simulink model "case7"  (R2024b)
settings: Solver=FixedStepAuto  StartTime=0  StopTime=1  FixedStep=1e-7  RelTol=1e-3
values from neighbouring files (symbols this model uses):
  SG_D_1_D = 0.01056    [IEEE9_case_parameters.m]    (also in case1_parameters.m; case2_parameters.m; case3_parameters.m; case4_parameters.m)
  SG_D_1_EnableSaturation = 0    [IEEE9_case_parameters.m]    (also in case1_parameters.m; case2_parameters.m; case3_parameters.m; case4_parameters.m)
  SG_D_1_f0 = 60    [IEEE9_case_parameters.m]    (also in case1_parameters.m; case2_parameters.m; case3_parameters.m; case4_parameters.m)
  SG_D_1_H = 7.5    [IEEE9_case_parameters.m]    (also in case1_parameters.m; case2_parameters.m; case3_parameters.m; case4_parameters.m)
  SG_D_1_K_A = 20    [IEEE9_case_parameters.m]    (also in case1_parameters.m; case2_parameters.m; case3_parameters.m; case4_parameters.m)
  SG_D_1_K_E = 1.000000e+1    (= 10)    [IEEE9_case_parameters.m]    (also in case1_parameters.m; case2_parameters.m; case3_parameters.m; case4_parameters.m)
  SG_D_1_K_F = 2.363    [IEEE9_case_parameters.m]    (also in case1_parameters.m; case2_parameters.m; case3_parameters.m; case4_parameters.m)
  SG_D_1_K_s = 0.5    [IEEE9_case_parameters.m]    (also in case1_parameters.m = 5; case2_parameters.m = 5; case3_parameters.m = 5; case4_parameters.m = 5)
  SG_D_1_R_a = 0.001088    [IEEE9_case_parameters.m]    (also in case1_parameters.m; case2_parameters.m; case3_parameters.m; case4_parameters.m)
  SG_D_1_S_A = 1    [IEEE9_case_parameters.m]    (also in case1_parameters.m; case2_parameters.m; case3_parameters.m; case4_parameters.m)
  SG_D_1_S_B = 0.103    [IEEE9_case_parameters.m]    (also in case1_parameters.m; case2_parameters.m; case3_parameters.m; case4_parameters.m)
  SG_D_1_S_N = 10.659857    [IEEE9_case_parameters.m]    (also in case1_parameters.m; case2_parameters.m; case3_parameters.m; case4_parameters.m)
  SG_D_1_SpeedPara = 200    [IEEE9_case_parameters.m]    (also in case1_parameters.m; case2_parameters.m; case3_parameters.m; case4_parameters.m)
  SG_D_1_T_0 = 0.720173    [IEEE9_case_parameters.m]    (also in case1_parameters.m = 0.755522; case2_parameters.m = 0.808931; case3_parameters.m = 0.869402; case4_parameters.m = 0.729316)
  SG_D_1_T_1 = 0.3    [IEEE9_case_parameters.m]    (also in case1_parameters.m; case2_parameters.m; case3_parameters.m; case4_parameters.m)
  SG_D_1_T_2 = 0.05    [IEEE9_case_parameters.m]    (also in case1_parameters.m; case2_parameters.m; case3_parameters.m; case4_parameters.m)
  SG_D_1_T_3 = 0.02    [IEEE9_case_parameters.m]    (also in case1_parameters.m; case2_parameters.m; case3_parameters.m; case4_parameters.m)
  SG_D_1_T_4 = 0.005    [IEEE9_case_parameters.m]    (also in case1_parameters.m; case2_parameters.m; case3_parameters.m; case4_parameters.m)
  SG_D_1_T_A = 0.02    [IEEE9_case_parameters.m]    (also in case1_parameters.m; case2_parameters.m; case3_parameters.m; case4_parameters.m)
  SG_D_1_T_dd = 8.000000e+0    (= 8)    [IEEE9_case_parameters.m]    (also in case1_parameters.m; case2_parameters.m; case3_parameters.m; case4_parameters.m)
  SG_D_1_T_ddd = 0.04    [IEEE9_case_parameters.m]    (also in case1_parameters.m; case2_parameters.m; case3_parameters.m; case4_parameters.m)
  SG_D_1_T_E = 0.314    [IEEE9_case_parameters.m]    (also in case1_parameters.m; case2_parameters.m; case3_parameters.m; case4_parameters.m)
  SG_D_1_T_F = 0.35    [IEEE9_case_parameters.m]    (also in case1_parameters.m; case2_parameters.m; case3_parameters.m; case4_parameters.m)
  SG_D_1_T_qd = 0.8    [IEEE9_case_parameters.m]    (also in case1_parameters.m; case2_parameters.m; case3_parameters.m; case4_parameters.m)
  SG_D_1_T_qdd = 0.02    [IEEE9_case_parameters.m]    (also in case1_parameters.m; case2_parameters.m; case3_parameters.m; case4_parameters.m)
  SG_D_1_T_speed = 0.1    [IEEE9_case_parameters.m]    (also in case1_parameters.m = 200; case2_parameters.m = 200; case3_parameters.m = 200; case4_parameters.m = 200)
  SG_D_1_T_w = 0.5    [IEEE9_case_parameters.m]    (also in case1_parameters.m; case2_parameters.m; case3_parameters.m; case4_parameters.m)
  SG_D_1_V_ref = 1.990276    [IEEE9_case_parameters.m]    (also in case1_parameters.m = 2.042296; case2_parameters.m = 2.051388; case3_parameters.m = 2.089584; case4_parameters.m = 2.01845)
  SG_D_1_w_ref = 376.991118    [IEEE9_case_parameters.m]    (also in case1_parameters.m; case2_parameters.m; case3_parameters.m; case4_parameters.m)
  SG_D_1_wb = 6.000000e+1    (= 60)    [IEEE9_case_parameters.m]    (also in case1_parameters.m; case2_parameters.m; case3_parameters.m; case4_parameters.m)
  SG_D_1_x_d = 1.9    [IEEE9_case_parameters.m]    (also in case1_parameters.m; case2_parameters.m; case3_parameters.m; case4_parameters.m)
  SG_D_1_x_dd = 0.302    [IEEE9_case_parameters.m]    (also in case1_parameters.m; case2_parameters.m; case3_parameters.m; case4_parameters.m)
  SG_D_1_x_ddd = 0.204    [IEEE9_case_parameters.m]    (also in case1_parameters.m; case2_parameters.m; case3_parameters.m; case4_parameters.m)
  SG_D_1_x_l = 0.05    [IEEE9_case_parameters.m]    (also in case1_parameters.m; case2_parameters.m; case3_parameters.m; case4_parameters.m)
  SG_D_1_x_q = 1.3    [IEEE9_case_parameters.m]    (also in case1_parameters.m; case2_parameters.m; case3_parameters.m; case4_parameters.m)
  SG_D_1_x_qd = 0.5    [IEEE9_case_parameters.m]    (also in case1_parameters.m; case2_parameters.m; case3_parameters.m; case4_parameters.m)
  SG_D_1_x_qdd = 0.3    [IEEE9_case_parameters.m]    (also in case1_parameters.m; case2_parameters.m; case3_parameters.m; case4_parameters.m)
  SG_D_2_D = 0.02    [IEEE9_case_parameters.m]    (also in case1_parameters.m; case2_parameters.m; case3_parameters.m; case4_parameters.m)
  SG_D_2_EnableSaturation = 0    [IEEE9_case_parameters.m]    (also in case1_parameters.m; case2_parameters.m; case3_parameters.m; case4_parameters.m)
  SG_D_2_f0 = 60    [IEEE9_case_parameters.m]    (also in case1_parameters.m; case2_parameters.m; case3_parameters.m; case4_parameters.m)
  SG_D_2_H = 8.000000e+0    (= 8)    [IEEE9_case_parameters.m]    (also in case1_parameters.m; case2_parameters.m; case3_parameters.m; case4_parameters.m)
  SG_D_2_K_A = 20    [IEEE9_case_parameters.m]    (also in case1_parameters.m; case2_parameters.m; case3_parameters.m; case4_parameters.m)
  SG_D_2_K_E = 1.000000e+1    (= 10)    [IEEE9_case_parameters.m]    (also in case1_parameters.m; case2_parameters.m; case3_parameters.m; case4_parameters.m)
  SG_D_2_K_F = 2.363    [IEEE9_case_parameters.m]    (also in case1_parameters.m; case2_parameters.m; case3_parameters.m; case4_parameters.m)
  SG_D_2_K_s = 0.5    [IEEE9_case_parameters.m]    (also in case1_parameters.m = 4; case2_parameters.m = 4; case3_parameters.m = 4; case4_parameters.m = 4)
  SG_D_2_R_a = 0.001088    [IEEE9_case_parameters.m]    (also in case1_parameters.m; case2_parameters.m; case3_parameters.m; case4_parameters.m)
  SG_D_2_S_A = 1    [IEEE9_case_parameters.m]    (also in case1_parameters.m; case2_parameters.m; case3_parameters.m; case4_parameters.m)
  SG_D_2_S_B = 0.103    [IEEE9_case_parameters.m]    (also in case1_parameters.m; case2_parameters.m; case3_parameters.m; case4_parameters.m)
  SG_D_2_S_N = 10.659857    [IEEE9_case_parameters.m]    (also in case1_parameters.m; case2_parameters.m; case3_parameters.m; case4_parameters.m)
  SG_D_2_SpeedPara = 200    [IEEE9_case_parameters.m]    (also in case1_parameters.m; case2_parameters.m; case3_parameters.m; case4_parameters.m)
  SG_D_2_T_0 = 1.632913    [IEEE9_case_parameters.m]    (also in case1_parameters.m = 1.632925; case2_parameters.m = 1.632915; case3_parameters.m = 1.632914; case4_parameters.m = 1.632927)
  SG_D_2_T_1 = 0.2    [IEEE9_case_parameters.m]    (also in case1_parameters.m; case2_parameters.m; case3_parameters.m; case4_parameters.m)
  SG_D_2_T_2 = 0.05    [IEEE9_case_parameters.m]    (also in case1_parameters.m; case2_parameters.m; case3_parameters.m; case4_parameters.m)
  SG_D_2_T_3 = 0.02    [IEEE9_case_parameters.m]    (also in case1_parameters.m; case2_parameters.m; case3_parameters.m; case4_parameters.m)
  SG_D_2_T_4 = 0.005    [IEEE9_case_parameters.m]    (also in case1_parameters.m; case2_parameters.m; case3_parameters.m; case4_parameters.m)
  SG_D_2_T_A = 0.02    [IEEE9_case_parameters.m]    (also in case1_parameters.m; case2_parameters.m; case3_parameters.m; case4_parameters.m)
  SG_D_2_T_dd = 7.9    [IEEE9_case_parameters.m]    (also in case1_parameters.m; case2_parameters.m; case3_parameters.m; case4_parameters.m)
  SG_D_2_T_ddd = 0.04    [IEEE9_case_parameters.m]    (also in case1_parameters.m; case2_parameters.m; case3_parameters.m; case4_parameters.m)
  SG_D_2_T_E = 0.314    [IEEE9_case_parameters.m]    (also in case1_parameters.m; case2_parameters.m; case3_parameters.m; case4_parameters.m)
  SG_D_2_T_F = 0.35    [IEEE9_case_parameters.m]    (also in case1_parameters.m; case2_parameters.m; case3_parameters.m; case4_parameters.m)
  SG_D_2_T_qd = 0.8    [IEEE9_case_parameters.m]    (also in case1_parameters.m; case2_parameters.m; case3_parameters.m; case4_parameters.m)
  SG_D_2_T_qdd = 0.015    [IEEE9_case_parameters.m]    (also in case1_parameters.m; case2_parameters.m; case3_parameters.m; case4_parameters.m)
  SG_D_2_T_speed = 0.1    [IEEE9_case_parameters.m]    (also in case1_parameters.m = 150; case2_parameters.m = 150; case3_parameters.m = 150; case4_parameters.m = 150)
  SG_D_2_T_w = 0.35    [IEEE9_case_parameters.m]    (also in case1_parameters.m; case2_parameters.m; case3_parameters.m; case4_parameters.m)
  SG_D_2_V_ref = 2.58547    [IEEE9_case_parameters.m]    (also in case1_parameters.m = 2.597896; case2_parameters.m = 2.587136; case3_parameters.m = 2.586042; case4_parameters.m = 2.599679)
  SG_D_2_w_ref = 376.991118    [IEEE9_case_parameters.m]    (also in case1_parameters.m; case2_parameters.m; case3_parameters.m; case4_parameters.m)
  SG_D_2_wb = 6.000000e+1    (= 60)    [IEEE9_case_parameters.m]    (also in case1_parameters.m; case2_parameters.m; case3_parameters.m; case4_parameters.m)
  SG_D_2_x_d = 1.8    [IEEE9_case_parameters.m]    (also in case1_parameters.m; case2_parameters.m; case3_parameters.m; case4_parameters.m)
  SG_D_2_x_dd = 0.302    [IEEE9_case_parameters.m]    (also in case1_parameters.m; case2_parameters.m; case3_parameters.m; case4_parameters.m)
  SG_D_2_x_ddd = 0.204    [IEEE9_case_parameters.m]    (also in case1_parameters.m; case2_parameters.m; case3_parameters.m; case4_parameters.m)
  SG_D_2_x_l = 0.05    [IEEE9_case_parameters.m]    (also in case1_parameters.m; case2_parameters.m; case3_parameters.m; case4_parameters.m)
  SG_D_2_x_q = 1.25    [IEEE9_case_parameters.m]    (also in case1_parameters.m; case2_parameters.m; case3_parameters.m; case4_parameters.m)
  SG_D_2_x_qd = 0.5    [IEEE9_case_parameters.m]    (also in case1_parameters.m; case2_parameters.m; case3_parameters.m; case4_parameters.m)
  SG_D_2_x_qdd = 0.3    [IEEE9_case_parameters.m]    (also in case1_parameters.m; case2_parameters.m; case3_parameters.m; case4_parameters.m)
  SG_D_3_D = 0.02    [IEEE9_case_parameters.m]    (also in case1_parameters.m; case2_parameters.m; case3_parameters.m; case4_parameters.m)
  SG_D_3_EnableSaturation = 0    [IEEE9_case_parameters.m]    (also in case1_parameters.m; case2_parameters.m; case3_parameters.m; case4_parameters.m)
  SG_D_3_f0 = 60    [IEEE9_case_parameters.m]    (also in case1_parameters.m; case2_parameters.m; case3_parameters.m; case4_parameters.m)
  SG_D_3_H = 7.7    [IEEE9_case_parameters.m]    (also in case1_parameters.m; case2_parameters.m; case3_parameters.m; case4_parameters.m)
  SG_D_3_K_A = 20    [IEEE9_case_parameters.m]    (also in case1_parameters.m; case2_parameters.m; case3_parameters.m; case4_parameters.m)
  SG_D_3_K_E = 1.000000e+1    (= 10)    [IEEE9_case_parameters.m]    (also in case1_parameters.m; case2_parameters.m; case3_parameters.m; case4_parameters.m)
  SG_D_3_K_F = 2.363    [IEEE9_case_parameters.m]    (also in case1_parameters.m; case2_parameters.m; case3_parameters.m; case4_parameters.m)
  SG_D_3_K_s = 0.2    [IEEE9_case_parameters.m]    (also in case1_parameters.m = 2; case2_parameters.m = 2; case3_parameters.m = 2; case4_parameters.m = 2)
  SG_D_3_R_a = 0.001088    [IEEE9_case_parameters.m]    (also in case1_parameters.m; case2_parameters.m; case3_parameters.m; case4_parameters.m)
  SG_D_3_S_A = 1    [IEEE9_case_parameters.m]    (also in case1_parameters.m; case2_parameters.m; case3_parameters.m; case4_parameters.m)
  SG_D_3_S_B = 0.103    [IEEE9_case_parameters.m]    (also in case1_parameters.m; case2_parameters.m; case3_parameters.m; case4_parameters.m)
  SG_D_3_S_N = 10.659857    [IEEE9_case_parameters.m]    (also in case1_parameters.m; case2_parameters.m; case3_parameters.m; case4_parameters.m)
  SG_D_3_SpeedPara = 200    [IEEE9_case_parameters.m]    (also in case1_parameters.m; case2_parameters.m; case3_parameters.m; case4_parameters.m)
  SG_D_3_T_0 = 0.850788    [IEEE9_case_parameters.m]    (also in case1_parameters.m = 0.850786; case2_parameters.m = 0.850787; case3_parameters.m; case4_parameters.m = 0.850786)
  SG_D_3_T_1 = 0.2    [IEEE9_case_parameters.m]    (also in case1_parameters.m; case2_parameters.m; case3_parameters.m; case4_parameters.m)
  SG_D_3_T_2 = 0.05    [IEEE9_case_parameters.m]    (also in case1_parameters.m; case2_parameters.m; case3_parameters.m; case4_parameters.m)
  SG_D_3_T_3 = 0.02    [IEEE9_case_parameters.m]    (also in case1_parameters.m; case2_parameters.m; case3_parameters.m; case4_parameters.m)
  SG_D_3_T_4 = 0.005    [IEEE9_case_parameters.m]    (also in case1_parameters.m; case2_parameters.m; case3_parameters.m; case4_parameters.m)
  SG_D_3_T_A = 0.02    [IEEE9_case_parameters.m]    (also in case1_parameters.m; case2_parameters.m; case3_parameters.m; case4_parameters.m)
  SG_D_3_T_dd = 8.1    [IEEE9_case_parameters.m]    (also in case1_parameters.m; case2_parameters.m; case3_parameters.m; case4_parameters.m)
  SG_D_3_T_ddd = 0.04    [IEEE9_case_parameters.m]    (also in case1_parameters.m; case2_parameters.m; case3_parameters.m; case4_parameters.m)
  SG_D_3_T_E = 0.314    [IEEE9_case_parameters.m]    (also in case1_parameters.m; case2_parameters.m; case3_parameters.m; case4_parameters.m)
  SG_D_3_T_F = 0.35    [IEEE9_case_parameters.m]    (also in case1_parameters.m; case2_parameters.m; case3_parameters.m; case4_parameters.m)
  SG_D_3_T_qd = 0.8    [IEEE9_case_parameters.m]    (also in case1_parameters.m; case2_parameters.m; case3_parameters.m; case4_parameters.m)
  SG_D_3_T_qdd = 0.015    [IEEE9_case_parameters.m]    (also in case1_parameters.m; case2_parameters.m; case3_parameters.m; case4_parameters.m)
  SG_D_3_T_speed = 0.1    [IEEE9_case_parameters.m]    (also in case1_parameters.m = 180; case2_parameters.m = 180; case3_parameters.m = 180; case4_parameters.m = 180)
  SG_D_3_T_w = 0.4    [IEEE9_case_parameters.m]    (also in case1_parameters.m; case2_parameters.m; case3_parameters.m; case4_parameters.m)
  SG_D_3_V_ref = 1.892727    [IEEE9_case_parameters.m]    (also in case1_parameters.m = 1.906439; case2_parameters.m = 1.895535; case3_parameters.m = 1.892105; case4_parameters.m = 1.906598)
  SG_D_3_w_ref = 376.991118    [IEEE9_case_parameters.m]    (also in case1_parameters.m; case2_parameters.m; case3_parameters.m; case4_parameters.m)
  SG_D_3_wb = 6.000000e+1    (= 60)    [IEEE9_case_parameters.m]    (also in case1_parameters.m; case2_parameters.m; case3_parameters.m; case4_parameters.m)
  SG_D_3_x_d = 1.85    [IEEE9_case_parameters.m]    (also in case1_parameters.m; case2_parameters.m; case3_parameters.m; case4_parameters.m)
  SG_D_3_x_dd = 0.302    [IEEE9_case_parameters.m]    (also in case1_parameters.m; case2_parameters.m; case3_parameters.m; case4_parameters.m)
  SG_D_3_x_ddd = 0.204    [IEEE9_case_parameters.m]    (also in case1_parameters.m; case2_parameters.m; case3_parameters.m; case4_parameters.m)
  SG_D_3_x_l = 0.05    [IEEE9_case_parameters.m]    (also in case1_parameters.m; case2_parameters.m; case3_parameters.m; case4_parameters.m)
  SG_D_3_x_q = 1.2    [IEEE9_case_parameters.m]    (also in case1_parameters.m; case2_parameters.m; case3_parameters.m; case4_parameters.m)
  SG_D_3_x_qd = 0.5    [IEEE9_case_parameters.m]    (also in case1_parameters.m; case2_parameters.m; case3_parameters.m; case4_parameters.m)
  SG_D_3_x_qdd = 0.3    [IEEE9_case_parameters.m]    (also in case1_parameters.m; case2_parameters.m; case3_parameters.m; case4_parameters.m)
(part 8 of 12)

== system case7/SG_D_2/d_psi_d_SG_D_2_block ==
  note: d_psi_d_SG_D_2 in case7
      | $2\,\pi \,f_{0}\,\left(v_{d,\mathrm{SG},D,2}\,\sin\left(\theta _{\mathrm{SG},D,2}\right)-v_{q,\mathrm{SG},D,2}\,\cos\left(\theta _{\mathrm{SG},D,2}\right)+\frac{R_{a}\,\left(\frac{\psi _{\mathrm{1d},\mathrm{SG},D,2}\,\left(x_{\mathrm{dd}}-x_{\mathrm{ddd}}\right)}{x_{\mathrm{dd}}-x_{l}}-\psi _{d,\mathrm{SG},D,2}+\frac{\psi _{\mathrm{fd},\mathrm{SG},D,2}\,\left(x_{\mathrm{ddd}}-x_{l}\right)}{x_{\mathrm{dd}}-x_{l}}\right)}{x_{\mathrm{ddd}}}+\frac{\psi _{q,\mathrm{SG},D,2}\,w_{\mathrm{SG},D,2}}{2\,f_{0}\,\pi }\right)$
      | Automatically generated on 2025-10-31 19:24:13 .
  State_psi_1d_SG_D_2_39a46 : Inport
  State_psi_d_SG_D_2_1ecaf : Inport  Port=2
  State_psi_fd_SG_D_2_079ef : Inport  Port=3
  Input_v_d_SG_D_2_793e9 : Inport  Port=4
  State_theta_SG_D_2_659a4 : Inport  Port=5
  Input_v_q_SG_D_2_3f1f5 : Inport  Port=6
  State_theta_SG_D_2_bf2b8 : Inport  Port=7
  State_psi_q_SG_D_2_5b767 : Inport  Port=8
  State_w_SG_D_2_79fa8 : Inport  Port=9
  Add_7ecc8 : Sum
  Add_e3358 : Sum
  Constant_-1_a36bb : Constant  Value=-1
  Constant_-2.0_2be6d : Constant  Value=-2.0
  Constant_2.0_21041 : Constant  Value=2.0
  Constant_R_a_76e05 : Constant  Value=R_a
  Constant_f0_5a6e6 : Constant  Value=f0
  Constant_f0_79645 : Constant  Value=f0
  Constant_pi_17814 : Constant  Value=pi
  Constant_pi_76bd4 : Constant  Value=pi
  Constant_x_dd_7bff0 : Constant  Value=x_dd
  Constant_x_dd_a337d : Constant  Value=x_dd
  Constant_x_dd_eede7 : Constant  Value=x_dd
  Constant_x_ddd_258ca : Constant  Value=x_ddd
  Constant_x_ddd_66dd9 : Constant  Value=x_ddd
  Constant_x_ddd_943a6 : Constant  Value=x_ddd
  Constant_x_l_530d0 : Constant  Value=x_l
  Constant_x_l_bb6df : Constant  Value=x_l
  Constant_x_l_feec9 : Constant  Value=x_l
  Divide_1fae6 : Product  Inputs=*/
  Divide_220e3 : Product  Inputs=*/
  Divide_44642 : Product  Inputs=*/
  Divide_cfd66 : Product  Inputs=*/
  MathFunc_cos_16d27 : Trigonometry  Operator=cos
  MathFunc_sin_a6049 : Trigonometry
  Product_23ef9 : Product
  Product_25772 : Product
  Product_48247 : Product
  Product_4d9a3 : Product
  Product_755c6 : Product
  Product_9b95b : Product
  Product_ba3b4 : Product
  Product_bcfea : Product
  Product_dfe12 : Product
  Product_eb8de : Product
  Product_f8462 : Product
  Product_f9716 : Product
  Subtract_0500b : Sum  Inputs=+-
  Subtract_09b2b : Sum  Inputs=+-
  Subtract_9b36a : Sum  Inputs=+-
  Subtract_a4b38 : Sum  Inputs=+-
  Subtract_cdce1 : Sum  Inputs=+-
  Subtract_e3d11 : Sum  Inputs=+-
  Subtract_f32b6 : Sum  Inputs=+-
  Blockout_d_psi_d_SG_D_2_9d3b5 : Outport
  wires:
  MathFunc_sin_a6049/1 -> Product_f9716/2
  Constant_x_dd_a337d/1 -> Subtract_cdce1/1
  Constant_-1_a36bb/1 -> Product_eb8de/1
  Constant_x_l_bb6df/1 -> Subtract_cdce1/2
  State_psi_1d_SG_D_2_39a46/1 -> Product_eb8de/2
  Constant_f0_79645/1 -> Product_4d9a3/2
  Constant_2.0_21041/1 -> Product_25772/1
  Constant_x_l_530d0/1 -> Subtract_f32b6/2
  Constant_x_dd_7bff0/1 -> Subtract_09b2b/1
  Product_23ef9/1 -> Blockout_d_psi_d_SG_D_2_9d3b5/1
  Constant_pi_76bd4/1 -> Product_25772/2
  Constant_x_ddd_258ca/1 -> Subtract_09b2b/2
  Subtract_a4b38/1 -> Product_23ef9/2
  Product_eb8de/1 -> Product_f8462/1
  Product_25772/1 -> Product_dfe12/1
  Subtract_09b2b/1 -> Product_f8462/2
  Divide_220e3/1 -> Subtract_a4b38/2
  Constant_x_ddd_943a6/1 -> Subtract_0500b/1
  Constant_x_l_feec9/1 -> Subtract_0500b/2
  Product_f8462/1 -> Divide_44642/1
  Subtract_9b36a/1 -> Add_7ecc8/1
  Subtract_cdce1/1 -> Divide_44642/2
  State_psi_fd_SG_D_2_079ef/1 -> Product_755c6/1
  Subtract_0500b/1 -> Product_755c6/2
  Constant_x_dd_eede7/1 -> Subtract_f32b6/1
  Divide_44642/1 -> Add_e3358/1
  State_psi_d_SG_D_2_1ecaf/1 -> Add_e3358/2
  Product_755c6/1 -> Divide_1fae6/1
  Subtract_f32b6/1 -> Divide_1fae6/2
  Add_e3358/1 -> Subtract_e3d11/1
  Divide_1fae6/1 -> Subtract_e3d11/2
  Constant_R_a_76e05/1 -> Product_ba3b4/1
  Subtract_e3d11/1 -> Product_ba3b4/2
  Divide_cfd66/1 -> Subtract_9b36a/1
  State_theta_SG_D_2_659a4/1 -> MathFunc_sin_a6049/1
  Product_ba3b4/1 -> Divide_cfd66/1
  Constant_-2.0_2be6d/1 -> Product_9b95b/1
  Input_v_d_SG_D_2_793e9/1 -> Product_f9716/1
  Constant_x_ddd_66dd9/1 -> Divide_cfd66/2
  State_theta_SG_D_2_bf2b8/1 -> MathFunc_cos_16d27/1
  Product_4d9a3/1 -> Product_23ef9/1
  Product_f9716/1 -> Subtract_9b36a/2
  Product_9b95b/1 -> Product_4d9a3/1
  Input_v_q_SG_D_2_3f1f5/1 -> Product_bcfea/1
  MathFunc_cos_16d27/1 -> Product_bcfea/2
  State_psi_q_SG_D_2_5b767/1 -> Product_48247/1
  State_w_SG_D_2_79fa8/1 -> Product_48247/2
  Constant_f0_5a6e6/1 -> Product_dfe12/2
  Constant_pi_17814/1 -> Product_9b95b/2
  Product_bcfea/1 -> Add_7ecc8/2
  Product_48247/1 -> Divide_220e3/1
  Product_dfe12/1 -> Divide_220e3/2
  Add_7ecc8/1 -> Subtract_a4b38/1

== system case7/SG_D_2/d_psi_fd_SG_D_2_block ==
  note: d_psi_fd_SG_D_2 in case7
      | $-\frac{\psi _{\mathrm{fd},\mathrm{SG},D,2}-E_{\mathrm{fd},\mathrm{SG},D,2}+\left(x_{d}-x_{\mathrm{dd}}\right)\,\left(\frac{\frac{\psi _{\mathrm{1d},\mathrm{SG},D,2}\,\left(x_{\mathrm{dd}}-x_{\mathrm{ddd}}\right)}{x_{\mathrm{dd}}-x_{l}}-\psi _{d,\mathrm{SG},D,2}+\frac{\psi _{\mathrm{fd},\mathrm{SG},D,2}\,\left(x_{\mathrm{ddd}}-x_{l}\right)}{x_{\mathrm{dd}}-x_{l}}}{x_{\mathrm{ddd}}}-\frac{\left(x_{\mathrm{dd}}-x_{\mathrm{ddd}}\right)\,\left(\psi _{\mathrm{1d},\mathrm{SG},D,2}-\psi _{\mathrm{fd},\mathrm{SG},D,2}+\frac{\left(x_{\mathrm{dd}}-x_{l}\right)\,\left(\frac{\psi _{\mathrm{1d},\mathrm{SG},D,2}\,\left(x_{\mathrm{dd}}-x_{\mathrm{ddd}}\right)}{x_{\mathrm{dd}}-x_{l}}-\psi _{d,\mathrm{SG},D,2}+\frac{\psi _{\mathrm{fd},\mathrm{SG},D,2}\,\left(x_{\mathrm{ddd}}-x_{l}\right)}{x_{\mathrm{dd}}-x_{l}}\right)}{x_{\mathrm{ddd}}}\right)}{{\left(x_{\mathrm{dd}}-x_{l}\right)}^2}\right)}{T_{\mathrm{dd}}}$
      | Automatically generated on 2025-10-31 19:24:23 .
  State_E_fd_SG_D_2_6abd7 : Inport
  State_psi_fd_SG_D_2_c8c63 : Inport  Port=2
  State_psi_1d_SG_D_2_57e67 : Inport  Port=3
  State_psi_fd_SG_D_2_c9eab : Inport  Port=4
  State_psi_1d_SG_D_2_8d090 : Inport  Port=5
  State_psi_d_SG_D_2_c1fee : Inport  Port=6
  State_psi_fd_SG_D_2_d23df : Inport  Port=7
  State_psi_1d_SG_D_2_76ec9 : Inport  Port=8
  State_psi_d_SG_D_2_fe578 : Inport  Port=9
  State_psi_fd_SG_D_2_17d9a : Inport  Port=10
  Add_b6a63 : Sum
  Add_bc73e : Sum
  Constant_-1_301fb : Constant  Value=-1
  Constant_-1_47837 : Constant  Value=-1
  Constant_-1_74ac9 : Constant  Value=-1
  Constant_2.0_594b5 : Constant  Value=2.0
  Constant_T_dd_5d29a : Constant  Value=T_dd
  Constant_x_d_82a8b : Constant  Value=x_d
  Constant_x_dd_0b019 : Constant  Value=x_dd
  Constant_x_dd_16d2f : Constant  Value=x_dd
  Constant_x_dd_1873a : Constant  Value=x_dd
  Constant_x_dd_2edd1 : Constant  Value=x_dd
  Constant_x_dd_4ec4b : Constant  Value=x_dd
  Constant_x_dd_68cbf : Constant  Value=x_dd
  Constant_x_dd_6ba65 : Constant  Value=x_dd
  Constant_x_dd_83a6b : Constant  Value=x_dd
  Constant_x_dd_8802d : Constant  Value=x_dd
  Constant_x_dd_f94d9 : Constant  Value=x_dd
  Constant_x_ddd_0764f : Constant  Value=x_ddd
  Constant_x_ddd_3bc07 : Constant  Value=x_ddd
  Constant_x_ddd_47d13 : Constant  Value=x_ddd
  Constant_x_ddd_a7579 : Constant  Value=x_ddd
  Constant_x_ddd_b8eb8 : Constant  Value=x_ddd
  Constant_x_ddd_d1ce4 : Constant  Value=x_ddd
  Constant_x_ddd_fcbe0 : Constant  Value=x_ddd
  Constant_x_l_2e7ab : Constant  Value=x_l
  Constant_x_l_52dad : Constant  Value=x_l
  Constant_x_l_53a2b : Constant  Value=x_l
  Constant_x_l_6a635 : Constant  Value=x_l
  Constant_x_l_7c27b : Constant  Value=x_l
  Constant_x_l_ba540 : Constant  Value=x_l
  Constant_x_l_bff75 : Constant  Value=x_l
  Constant_x_l_ec901 : Constant  Value=x_l
  Divide_0b3aa : Product  Inputs=*/
  Divide_41c53 : Product  Inputs=*/
  Divide_60a2a : Product  Inputs=*/
  Divide_61c97 : Product  Inputs=*/
  Divide_6373b : Product  Inputs=*/
  Divide_934bc : Product  Inputs=*/
  Divide_98439 : Product  Inputs=*/
  Divide_b9119 : Product  Inputs=*/
  Power_3c096 : Math  Operator=pow
  Product_05c5d : Product
  Product_0d175 : Product
  Product_2ece7 : Product
  Product_3ce78 : Product
  Product_4041d : Product
  Product_6f20f : Product
  Product_7239c : Product
  Product_8a8b6 : Product
  Product_a518b : Product
  Product_e8c4e : Product
  Subtract_06d58 : Sum  Inputs=+-
  Subtract_13c27 : Sum  Inputs=+-
  Subtract_1c718 : Sum  Inputs=+-
  Subtract_20010 : Sum  Inputs=+-
  Subtract_347ee : Sum  Inputs=+-
  Subtract_3ab27 : Sum  Inputs=+-
  Subtract_4c79f : Sum  Inputs=+-
  Subtract_5ecbd : Sum  Inputs=+-
  Subtract_8cc1a : Sum  Inputs=+-
  Subtract_909f5 : Sum  Inputs=+-
  Subtract_987f0 : Sum  Inputs=+-
  Subtract_98dad : Sum  Inputs=+-
  Subtract_9f70b : Sum  Inputs=+-
  Subtract_a810f : Sum  Inputs=+-
  Subtract_a8741 : Sum  Inputs=+-
  Subtract_c0dfd : Sum  Inputs=+-
  Subtract_ce58e : Sum  Inputs=+-
  Subtract_f0c5b : Sum  Inputs=+-
  Subtract_fc7c8 : Sum  Inputs=+-
  Blockout_d_psi_fd_SG_D_2_d186f : Outport
  wires:
  Constant_x_dd_83a6b/1 -> Subtract_9f70b/1
  Constant_-1_301fb/1 -> Product_0d175/1
  Constant_x_l_bff75/1 -> Subtract_f0c5b/2
  Divide_934bc/1 -> Add_bc73e/1
  Subtract_98dad/1 -> Product_4041d/2
  Constant_x_l_52dad/1 -> Subtract_9f70b/2
  Product_4041d/1 -> Divide_61c97/1
  State_psi_1d_SG_D_2_8d090/1 -> Product_0d175/2
  Constant_x_dd_1873a/1 -> Subtract_20010/1
  Product_8a8b6/1 -> Divide_934bc/1
  Constant_x_dd_8802d/1 -> Subtract_4c79f/1
  Constant_x_ddd_fcbe0/1 -> Subtract_20010/2
  Constant_x_dd_68cbf/1 -> Subtract_3ab27/1
  Product_0d175/1 -> Product_05c5d/1
  Subtract_20010/1 -> Product_05c5d/2
  State_psi_d_SG_D_2_fe578/1 -> Add_bc73e/2
  Constant_x_ddd_47d13/1 -> Subtract_98dad/1
  Constant_x_l_ec901/1 -> Subtract_98dad/2
  Product_05c5d/1 -> Divide_60a2a/1
  Subtract_9f70b/1 -> Divide_60a2a/2
  State_psi_fd_SG_D_2_d23df/1 -> Product_4041d/1
  Subtract_347ee/1 -> Product_e8c4e/2
  Constant_x_dd_6ba65/1 -> Subtract_a810f/1
  Constant_x_l_ba540/1 -> Subtract_a810f/2
  Product_7239c/1 -> Product_e8c4e/1
  Divide_60a2a/1 -> Add_b6a63/1
  State_psi_d_SG_D_2_c1fee/1 -> Add_b6a63/2
  Subtract_a810f/1 -> Divide_61c97/2
  Constant_x_dd_16d2f/1 -> Subtract_f0c5b/1
  Constant_x_ddd_d1ce4/1 -> Subtract_5ecbd/1
  Add_b6a63/1 -> Subtract_13c27/1
  Divide_61c97/1 -> Subtract_13c27/2
  Constant_-1_74ac9/1 -> Product_6f20f/1
  Product_2ece7/1 -> Divide_41c53/1
  State_psi_1d_SG_D_2_76ec9/1 -> Product_6f20f/2
  Subtract_4c79f/1 -> Product_7239c/2
  Constant_x_dd_f94d9/1 -> Subtract_c0dfd/1
  Divide_41c53/1 -> Subtract_06d58/2
  Constant_-1_47837/1 -> Product_7239c/1
  Constant_x_ddd_b8eb8/1 -> Subtract_c0dfd/2
  Constant_x_ddd_a7579/1 -> Divide_b9119/2
  Subtract_f0c5b/1 -> Product_a518b/1
  Subtract_13c27/1 -> Product_a518b/2
  State_psi_fd_SG_D_2_c9eab/1 -> Subtract_8cc1a/2
  Product_6f20f/1 -> Product_8a8b6/1
  Subtract_c0dfd/1 -> Product_8a8b6/2
  Constant_2.0_594b5/1 -> Power_3c096/2
  State_psi_1d_SG_D_2_57e67/1 -> Subtract_8cc1a/1
  Constant_x_dd_2edd1/1 -> Subtract_1c718/1
  Subtract_5ecbd/1 -> Product_2ece7/2
  Constant_x_l_6a635/1 -> Subtract_1c718/2
  Constant_x_l_2e7ab/1 -> Subtract_5ecbd/2
  Constant_x_ddd_0764f/1 -> Subtract_4c79f/2
  Subtract_3ab27/1 -> Divide_41c53/2
  Product_a518b/1 -> Divide_b9119/1
  Subtract_1c718/1 -> Divide_934bc/2
  State_psi_fd_SG_D_2_17d9a/1 -> Product_2ece7/1
  Constant_x_l_53a2b/1 -> Subtract_3ab27/2
  Constant_x_dd_4ec4b/1 -> Subtract_ce58e/1
  Subtract_8cc1a/1 -> Subtract_347ee/1
  Divide_b9119/1 -> Subtract_347ee/2
  Constant_x_l_7c27b/1 -> Subtract_ce58e/2
  Subtract_ce58e/1 -> Power_3c096/1
  Add_bc73e/1 -> Subtract_06d58/1
  Product_e8c4e/1 -> Divide_6373b/1
  Power_3c096/1 -> Divide_6373b/2
  Subtract_06d58/1 -> Divide_98439/1
  Constant_x_ddd_3bc07/1 -> Divide_98439/2
  Constant_x_d_82a8b/1 -> Subtract_909f5/1
  Constant_x_dd_0b019/1 -> Subtract_909f5/2
  Divide_6373b/1 -> Subtract_987f0/1
  Divide_98439/1 -> Subtract_987f0/2
  State_E_fd_SG_D_2_6abd7/1 -> Subtract_a8741/1
  State_psi_fd_SG_D_2_c8c63/1 -> Subtract_a8741/2
  Subtract_909f5/1 -> Product_3ce78/1
  Subtract_987f0/1 -> Product_3ce78/2
  Subtract_a8741/1 -> Subtract_fc7c8/1
  Product_3ce78/1 -> Subtract_fc7c8/2
  Subtract_fc7c8/1 -> Divide_0b3aa/1
  Constant_T_dd_5d29a/1 -> Divide_0b3aa/2
  Divide_0b3aa/1 -> Blockout_d_psi_fd_SG_D_2_d186f/1

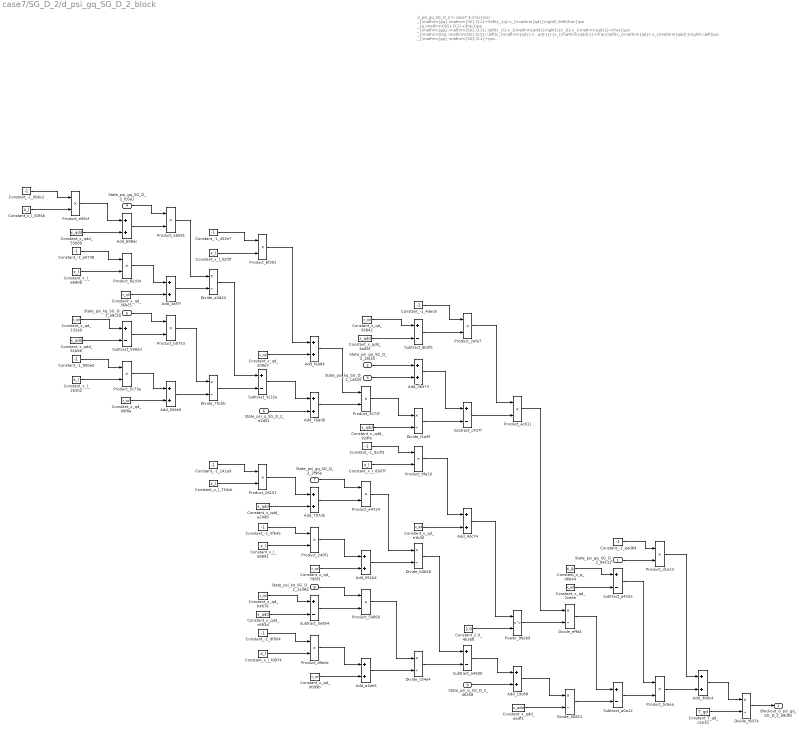
== system case7/SG_D_2/d_psi_gq_SG_D_2_block ==
  note: d_psi_gq_SG_D_2 in case7
      | $-\frac{\psi _{\mathrm{gq},\mathrm{SG},D,2}+\left(x_{q}-x_{\mathrm{qd}}\right)\,\left(\frac{\psi _{q,\mathrm{SG},D,2}+\frac{\psi _{\mathrm{gq},\mathrm{SG},D,2}\,\left(x_{l}-x_{\mathrm{qdd}}\right)}{x_{l}-x_{\mathrm{qd}}}+\frac{\psi _{\mathrm{kq},\mathrm{SG},D,2}\,\left(x_{\mathrm{qd}}-x_{\mathrm{qdd}}\right)}{x_{l}-x_{\mathrm{qd}}}}{x_{\mathrm{qdd}}}+\frac{\left(x_{\mathrm{qd}}-x_{\mathrm{qdd}}\right)\,\left(\psi _{\mathrm{gq},\mathrm{SG},D,2}+\psi _{\mathrm{kq},\mathrm{SG},D,2}+\frac{\left(x_{l}-x_{\mathrm{qd}}\right)\,\left(\psi _{q,\mathrm{SG},D,2}+\frac{\psi _{\mathrm{gq},\mathrm{SG},D,2}\,\left(x_{l}-x_{\mathrm{qdd}}\right)}{x_{l}-x_{\mathrm{qd}}}+\frac{\psi _{\mathrm{kq},\mathrm{SG},D,2}\,\left(x_{\mathrm{qd}}-x_{\mathrm{qdd}}\right)}{x_{l}-x_{\mathrm{qd}}}\right)}{x_{\mathrm{qdd}}}\right)}{{\left(x_{l}-x_{\mathrm{qd}}\right)}^2}\right)}{T_{\mathrm{qd}}}$
      | Automatically generated on 2025-10-31 19:24:34 .
  State_psi_gq_SG_D_2_04112 : Inport
  State_psi_gq_SG_D_2_2f535 : Inport  Port=2
  State_psi_kq_SG_D_2_14835 : Inport  Port=3
  State_psi_gq_SG_D_2_fc0a1 : Inport  Port=4
  State_psi_kq_SG_D_2_a8c2a : Inport  Port=5
  State_psi_q_SG_D_2_e2d01 : Inport  Port=6
  State_psi_gq_SG_D_2_2f96e : Inport  Port=7
  State_psi_kq_SG_D_2_1a38a : Inport  Port=8
  State_psi_q_SG_D_2_46358 : Inport  Port=9
  Add_051b4 : Sum
  Add_19c88 : Sum
  Add_369c4 : Sum
  Add_3b373 : Sum
  Add_43c74 : Sum
  Add_4af7f : Sum
  Add_504e5 : Sum
  Add_608ac : Sum
  Add_707d5 : Sum
  Add_76ad6 : Sum
  Add_a3de5 : Sum
  Add_feb84 : Sum
  Constant_-1_0b6c2 : Constant  Value=-1
  Constant_-1_241a9 : Constant  Value=-1
  Constant_-1_452e7 : Constant  Value=-1
  Constant_-1_4dec8 : Constant  Value=-1
  Constant_-1_5fb45 : Constant  Value=-1
  Constant_-1_900e0 : Constant  Value=-1
  Constant_-1_9cdf3 : Constant  Value=-1
  Constant_-1_df004 : Constant  Value=-1
  Constant_-1_e0738 : Constant  Value=-1
  Constant_-1_eed84 : Constant  Value=-1
  Constant_2.0_4b3b8 : Constant  Value=2.0
  Constant_T_qd_c5a1d : Constant  Value=T_qd
  Constant_x_l_02f0f : Constant  Value=x_l
  Constant_x_l_09d7f : Constant  Value=x_l
  Constant_x_l_2b3b2 : Constant  Value=x_l
  Constant_x_l_56891 : Constant  Value=x_l
  Constant_x_l_734cb : Constant  Value=x_l
  Constant_x_l_83f4b : Constant  Value=x_l
  Constant_x_l_e6906 : Constant  Value=x_l
  Constant_x_l_fd974 : Constant  Value=x_l
  Constant_x_q_d6b44 : Constant  Value=x_q
  Constant_x_qd_06f8a : Constant  Value=x_qd
  Constant_x_qd_132a0 : Constant  Value=x_qd
  Constant_x_qd_208e3 : Constant  Value=x_qd
  Constant_x_qd_2ceeb : Constant  Value=x_qd
  Constant_x_qd_36bc5 : Constant  Value=x_qd
  Constant_x_qd_56842 : Constant  Value=x_qd
  Constant_x_qd_796f3 : Constant  Value=x_qd
  Constant_x_qd_9099b : Constant  Value=x_qd
  Constant_x_qd_b4676 : Constant  Value=x_qd
  Constant_x_qd_e1b30 : Constant  Value=x_qd
  Constant_x_qdd_4a06f : Constant  Value=x_qdd
  Constant_x_qdd_55b09 : Constant  Value=x_qdd
  Constant_x_qdd_61b66 : Constant  Value=x_qdd
  Constant_x_qdd_92dfe : Constant  Value=x_qdd
  Constant_x_qdd_a24d8 : Constant  Value=x_qdd
  Constant_x_qdd_c693d : Constant  Value=x_qdd
  Constant_x_qdd_eadf1 : Constant  Value=x_qdd
  Divide_00821 : Product  Inputs=*/
  Divide_64b58 : Product  Inputs=*/
  Divide_75cbb : Product  Inputs=*/
  Divide_a3d24 : Product  Inputs=*/
  Divide_c54e4 : Product  Inputs=*/
  Divide_effd4 : Product  Inputs=*/
  Divide_f1a8f : Product  Inputs=*/
  Divide_f8374 : Product  Inputs=*/
  Power_96eb9 : Math  Operator=pow
  Product_240f1 : Product
  Product_26151 : Product
  Product_2efa7 : Product
  Product_3571f : Product
  Product_54860 : Product
  Product_5c6ea : Product
  Product_5c73a : Product
  Product_6f391 : Product
  Product_82c04 : Product
  Product_9fa10 : Product
  Product_ac911 : Product
  Product_b9753 : Product
  Product_d1e13 : Product
  Product_d9edc : Product
  Product_e09cf : Product
  Product_e4724 : Product
  Product_eb691 : Product
  Subtract_3c22e : Sum  Inputs=+-
  Subtract_5992d : Sum  Inputs=+-
  Subtract_5e854 : Sum  Inputs=+-
  Subtract_6b0f5 : Sum  Inputs=+-
  Subtract_a0a12 : Sum  Inputs=+-
  Subtract_a432e : Sum  Inputs=+-
  Subtract_a4500 : Sum  Inputs=+-
  Subtract_c437f : Sum  Inputs=+-
  Blockout_d_psi_gq_SG_D_2_e8d92 : Outport
  wires:
  Constant_x_l_fd974/1 -> Product_d9edc/2
  Constant_x_l_734cb/1 -> Product_26151/2
  Constant_x_qd_132a0/1 -> Subtract_5992d/1
  Constant_x_l_09d7f/1 -> Product_9fa10/2
  Constant_x_qdd_4a06f/1 -> Subtract_6b0f5/2
  Constant_-1_900e0/1 -> Product_5c73a/1
  Constant_-1_0b6c2/1 -> Product_e09cf/1
  State_psi_gq_SG_D_2_2f535/1 -> Add_3b373/1
  Constant_x_qdd_61b66/1 -> Subtract_5992d/2
  Constant_x_qd_56842/1 -> Subtract_6b0f5/1
  Constant_x_l_2b3b2/1 -> Product_5c73a/2
  Constant_x_l_83f4b/1 -> Product_e09cf/2
  Product_5c73a/1 -> Add_504e5/1
  Product_e09cf/1 -> Add_608ac/1
  Constant_x_l_e6906/1 -> Product_82c04/2
  Constant_x_l_02f0f/1 -> Product_6f391/2
  Constant_x_qd_06f8a/1 -> Add_504e5/2
  Constant_x_qdd_55b09/1 -> Add_608ac/2
  Constant_-1_e0738/1 -> Product_82c04/1
  Constant_x_qd_9099b/1 -> Add_a3de5/2
  Constant_x_qdd_a24d8/1 -> Add_707d5/2
  State_psi_gq_SG_D_2_fc0a1/1 -> Product_eb691/1
  Add_504e5/1 -> Divide_75cbb/2
  Add_608ac/1 -> Product_eb691/2
  Constant_x_qd_2ceeb/1 -> Subtract_a432e/2
  Product_82c04/1 -> Add_4af7f/1
  Constant_x_qd_36bc5/1 -> Add_4af7f/2
  State_psi_kq_SG_D_2_a8c2a/1 -> Product_b9753/1
  Divide_a3d24/1 -> Subtract_3c22e/1
  Subtract_5992d/1 -> Product_b9753/2
  Product_eb691/1 -> Divide_a3d24/1
  Add_4af7f/1 -> Divide_a3d24/2
  Add_76ad6/1 -> Product_3571f/2
  Product_b9753/1 -> Divide_75cbb/1
  Constant_-1_452e7/1 -> Product_6f391/1
  Divide_75cbb/1 -> Subtract_3c22e/2
  Constant_-1_df004/1 -> Product_d9edc/1
  Constant_-1_241a9/1 -> Product_26151/1
  Product_6f391/1 -> Add_feb84/1
  Constant_x_qdd_c693d/1 -> Subtract_5e854/2
  Constant_x_qd_208e3/1 -> Add_feb84/2
  Subtract_3c22e/1 -> Add_76ad6/1
  Constant_-1_9cdf3/1 -> Product_9fa10/1
  State_psi_q_SG_D_2_e2d01/1 -> Add_76ad6/2
  Product_d9edc/1 -> Add_a3de5/1
  Product_26151/1 -> Add_707d5/1
  Constant_-1_5fb45/1 -> Product_240f1/1
  Product_3571f/1 -> Divide_f1a8f/1
  Constant_x_l_56891/1 -> Product_240f1/2
  Product_5c6ea/1 -> Add_369c4/2
  Constant_x_qd_b4676/1 -> Subtract_5e854/1
  Add_feb84/1 -> Product_3571f/1
  State_psi_gq_SG_D_2_2f96e/1 -> Product_e4724/1
  Add_a3de5/1 -> Divide_c54e4/2
  Add_707d5/1 -> Product_e4724/2
  Product_240f1/1 -> Add_051b4/1
  Constant_x_qd_796f3/1 -> Add_051b4/2
  State_psi_kq_SG_D_2_1a38a/1 -> Product_54860/1
  Subtract_5e854/1 -> Product_54860/2
  Divide_c54e4/1 -> Subtract_a4500/2
  State_psi_kq_SG_D_2_14835/1 -> Add_3b373/2
  Product_54860/1 -> Divide_c54e4/1
  Constant_x_qdd_92dfe/1 -> Divide_f1a8f/2
  Product_e4724/1 -> Divide_64b58/1
  Add_051b4/1 -> Divide_64b58/2
  Constant_-1_4dec8/1 -> Product_2efa7/1
  Subtract_6b0f5/1 -> Product_2efa7/2
  Add_3b373/1 -> Subtract_c437f/1
  Divide_f1a8f/1 -> Subtract_c437f/2
  Product_9fa10/1 -> Add_43c74/1
  Constant_x_qd_e1b30/1 -> Add_43c74/2
  Divide_64b58/1 -> Subtract_a4500/1
  Product_2efa7/1 -> Product_ac911/1
  Subtract_c437f/1 -> Product_ac911/2
  Add_43c74/1 -> Power_96eb9/1
  Constant_2.0_4b3b8/1 -> Power_96eb9/2
  Subtract_a4500/1 -> Add_19c88/1
  State_psi_q_SG_D_2_46358/1 -> Add_19c88/2
  Product_ac911/1 -> Divide_effd4/1
  Power_96eb9/1 -> Divide_effd4/2
  Add_19c88/1 -> Divide_00821/1
  Constant_x_qdd_eadf1/1 -> Divide_00821/2
  Constant_x_q_d6b44/1 -> Subtract_a432e/1
  Divide_effd4/1 -> Subtract_a0a12/1
  Divide_00821/1 -> Subtract_a0a12/2
  Divide_f8374/1 -> Blockout_d_psi_gq_SG_D_2_e8d92/1
  Constant_-1_eed84/1 -> Product_d1e13/1
  State_psi_gq_SG_D_2_04112/1 -> Product_d1e13/2
  Subtract_a432e/1 -> Product_5c6ea/1
  Subtract_a0a12/1 -> Product_5c6ea/2
  Product_d1e13/1 -> Add_369c4/1
  Add_369c4/1 -> Divide_f8374/1
  Constant_T_qd_c5a1d/1 -> Divide_f8374/2

== system case7/SG_D_2/d_psi_kq_SG_D_2_block ==
  note: d_psi_kq_SG_D_2 in case7
      | $-\frac{\psi _{\mathrm{gq},\mathrm{SG},D,2}+\psi _{\mathrm{kq},\mathrm{SG},D,2}+\frac{\left(x_{l}-x_{\mathrm{qd}}\right)\,\left(\psi _{q,\mathrm{SG},D,2}+\frac{\psi _{\mathrm{gq},\mathrm{SG},D,2}\,\left(x_{l}-x_{\mathrm{qdd}}\right)}{x_{l}-x_{\mathrm{qd}}}+\frac{\psi _{\mathrm{kq},\mathrm{SG},D,2}\,\left(x_{\mathrm{qd}}-x_{\mathrm{qdd}}\right)}{x_{l}-x_{\mathrm{qd}}}\right)}{x_{\mathrm{qdd}}}}{T_{\mathrm{qdd}}}$
      | Automatically generated on 2025-10-31 19:24:38 .
  State_psi_gq_SG_D_2_30603 : Inport
  State_psi_kq_SG_D_2_1ae2e : Inport  Port=2
  State_psi_gq_SG_D_2_ebfa7 : Inport  Port=3
  State_psi_kq_SG_D_2_d9628 : Inport  Port=4
  State_psi_q_SG_D_2_5421a : Inport  Port=5
  Add_03404 : Sum
  Add_053de : Sum
  Add_1e86d : Sum
  Add_51960 : Sum
  Add_5f7ee : Sum
  Add_7df19 : Sum
  Constant_-1_63958 : Constant  Value=-1
  Constant_-1_aafbe : Constant  Value=-1
  Constant_-1_d98d5 : Constant  Value=-1
  Constant_-1_df802 : Constant  Value=-1
  Constant_-1_fafab : Constant  Value=-1
  Constant_T_qdd_74f44 : Constant  Value=T_qdd
  Constant_x_l_8fd93 : Constant  Value=x_l
  Constant_x_l_bf778 : Constant  Value=x_l
  Constant_x_l_c3542 : Constant  Value=x_l
  Constant_x_l_e7627 : Constant  Value=x_l
  Constant_x_qd_893d6 : Constant  Value=x_qd
  Constant_x_qd_d446d : Constant  Value=x_qd
  Constant_x_qd_e2da0 : Constant  Value=x_qd
  Constant_x_qd_fdc3b : Constant  Value=x_qd
  Constant_x_qdd_1cb1d : Constant  Value=x_qdd
  Constant_x_qdd_d7928 : Constant  Value=x_qdd
  Constant_x_qdd_f9e1c : Constant  Value=x_qdd
  Divide_24203 : Product  Inputs=*/
  Divide_41d1d : Product  Inputs=*/
  Divide_53881 : Product  Inputs=*/
  Divide_f75cf : Product  Inputs=*/
  Product_06998 : Product
  Product_4101a : Product
  Product_5794f : Product
  Product_7f224 : Product
  Product_ad00b : Product
  Product_e81ac : Product
  Product_efe8e : Product
  Product_f7369 : Product
  Subtract_22307 : Sum  Inputs=+-
  Subtract_c2b67 : Sum  Inputs=+-
  Subtract_dd147 : Sum  Inputs=+-
  Blockout_d_psi_kq_SG_D_2_9fcf6 : Outport
  wires:
  State_psi_kq_SG_D_2_1ae2e/1 -> Subtract_dd147/2
  Constant_-1_aafbe/1 -> Product_e81ac/1
  Constant_-1_fafab/1 -> Product_5794f/1
  Constant_x_l_c3542/1 -> Product_5794f/2
  Constant_x_qdd_1cb1d/1 -> Add_7df19/2
  Constant_x_l_8fd93/1 -> Product_e81ac/2
  Constant_x_qd_e2da0/1 -> Subtract_22307/1
  Constant_T_qdd_74f44/1 -> Divide_53881/2
  Constant_-1_63958/1 -> Product_efe8e/1
  Product_5794f/1 -> Add_7df19/1
  Constant_x_qdd_f9e1c/1 -> Subtract_22307/2
  Constant_x_l_e7627/1 -> Product_efe8e/2
  Divide_53881/1 -> Blockout_d_psi_kq_SG_D_2_9fcf6/1
  State_psi_gq_SG_D_2_ebfa7/1 -> Product_4101a/1
  Add_7df19/1 -> Product_4101a/2
  Product_e81ac/1 -> Add_5f7ee/1
  Constant_x_qd_fdc3b/1 -> Add_5f7ee/2
  Product_ad00b/1 -> Divide_41d1d/1
  State_psi_kq_SG_D_2_d9628/1 -> Product_7f224/1
  Subtract_22307/1 -> Product_7f224/2
  Product_efe8e/1 -> Add_1e86d/1
  Constant_x_qd_893d6/1 -> Add_1e86d/2
  Product_7f224/1 -> Divide_24203/1
  Product_4101a/1 -> Divide_f75cf/1
  Add_5f7ee/1 -> Divide_f75cf/2
  Add_1e86d/1 -> Divide_24203/2
  State_psi_q_SG_D_2_5421a/1 -> Add_03404/2
  Constant_-1_d98d5/1 -> Product_f7369/1
  Constant_x_l_bf778/1 -> Product_f7369/2
  Divide_f75cf/1 -> Subtract_c2b67/1
  Divide_24203/1 -> Subtract_c2b67/2
  Product_f7369/1 -> Add_053de/1
  Constant_x_qd_d446d/1 -> Add_053de/2
  Subtract_c2b67/1 -> Add_03404/1
  Constant_x_qdd_d7928/1 -> Divide_41d1d/2
  Constant_-1_df802/1 -> Product_06998/1
  State_psi_gq_SG_D_2_30603/1 -> Product_06998/2
  Add_053de/1 -> Product_ad00b/1
  Add_03404/1 -> Product_ad00b/2
  Product_06998/1 -> Subtract_dd147/1
  Subtract_dd147/1 -> Add_51960/1
  Divide_41d1d/1 -> Add_51960/2
  Add_51960/1 -> Divide_53881/1

== system case7/SG_D_2/d_psi_q_SG_D_2_block ==
  note: d_psi_q_SG_D_2 in case7
      | $2\,\pi \,f_{0}\,\left(v_{d,\mathrm{SG},D,2}\,\cos\left(\theta _{\mathrm{SG},D,2}\right)+v_{q,\mathrm{SG},D,2}\,\sin\left(\theta _{\mathrm{SG},D,2}\right)-\frac{R_{a}\,\left(\psi _{q,\mathrm{SG},D,2}+\frac{\psi _{\mathrm{gq},\mathrm{SG},D,2}\,\left(x_{l}-x_{\mathrm{qdd}}\right)}{x_{l}-x_{\mathrm{qd}}}+\frac{\psi _{\mathrm{kq},\mathrm{SG},D,2}\,\left(x_{\mathrm{qd}}-x_{\mathrm{qdd}}\right)}{x_{l}-x_{\mathrm{qd}}}\right)}{x_{\mathrm{qdd}}}-\frac{\psi _{d,\mathrm{SG},D,2}\,w_{\mathrm{SG},D,2}}{2\,f_{0}\,\pi }\right)$
      | Automatically generated on 2025-10-31 19:24:17 .
  State_psi_gq_SG_D_2_7156c : Inport
  State_psi_kq_SG_D_2_21fa1 : Inport  Port=2
  State_psi_q_SG_D_2_91656 : Inport  Port=3
  Input_v_d_SG_D_2_12f1d : Inport  Port=4
  State_theta_SG_D_2_c47ee : Inport  Port=5
  Input_v_q_SG_D_2_7d1d1 : Inport  Port=6
  State_theta_SG_D_2_7c757 : Inport  Port=7
  State_psi_d_SG_D_2_b6b26 : Inport  Port=8
  State_w_SG_D_2_933ea : Inport  Port=9
  Add_4d1a4 : Sum
  Add_65cf9 : Sum
  Add_79dd5 : Sum
  Add_7b5f3 : Sum
  Add_bfdbe : Sum
  Constant_-1_027eb : Constant  Value=-1
  Constant_-1_5db2a : Constant  Value=-1
  Constant_-1_e8c37 : Constant  Value=-1
  Constant_-2.0_8dfc0 : Constant  Value=-2.0
  Constant_2.0_eef07 : Constant  Value=2.0
  Constant_R_a_e4cab : Constant  Value=R_a
  Constant_f0_35b52 : Constant  Value=f0
  Constant_f0_6845f : Constant  Value=f0
  Constant_pi_184e6 : Constant  Value=pi
  Constant_pi_bbed2 : Constant  Value=pi
  Constant_x_l_2040c : Constant  Value=x_l
  Constant_x_l_8059f : Constant  Value=x_l
  Constant_x_l_d9db2 : Constant  Value=x_l
  Constant_x_qd_76623 : Constant  Value=x_qd
  Constant_x_qd_bdcc5 : Constant  Value=x_qd
  Constant_x_qd_faa1b : Constant  Value=x_qd
  Constant_x_qdd_0a686 : Constant  Value=x_qdd
  Constant_x_qdd_674d6 : Constant  Value=x_qdd
  Constant_x_qdd_72180 : Constant  Value=x_qdd
  Divide_254b3 : Product  Inputs=*/
  Divide_28f81 : Product  Inputs=*/
  Divide_60bc7 : Product  Inputs=*/
  Divide_7a6f1 : Product  Inputs=*/
  MathFunc_cos_c1fb4 : Trigonometry  Operator=cos
  MathFunc_sin_84ebb : Trigonometry
  Product_08807 : Product
  Product_0e53f : Product
  Product_2186e : Product
  Product_2d533 : Product
  Product_33a49 : Product
  Product_4159f : Product
  Product_4e2f0 : Product
  Product_6482a : Product
  Product_74126 : Product
  Product_7677e : Product
  Product_a70f7 : Product
  Product_a83a1 : Product
  Product_e911c : Product
  Product_f57b2 : Product
  Subtract_52d26 : Sum  Inputs=+-
  Subtract_651ed : Sum  Inputs=+-
  Subtract_9953e : Sum  Inputs=+-
  Subtract_e9756 : Sum  Inputs=+-
  Blockout_d_psi_q_SG_D_2_62d90 : Outport
  wires:
  Constant_x_qdd_0a686/1 -> Subtract_9953e/2
  Constant_x_l_8059f/1 -> Product_e911c/2
  Constant_-1_027eb/1 -> Product_6482a/1
  Constant_x_l_2040c/1 -> Product_6482a/2
  Product_6482a/1 -> Add_65cf9/1
  Constant_pi_bbed2/1 -> Product_7677e/2
  State_psi_gq_SG_D_2_7156c/1 -> Product_a83a1/1
  Constant_x_l_d9db2/1 -> Product_08807/2
  State_w_SG_D_2_933ea/1 -> Product_2186e/2
  Constant_x_qd_faa1b/1 -> Add_79dd5/2
  Constant_x_qdd_674d6/1 -> Add_65cf9/2
  Constant_2.0_eef07/1 -> Product_7677e/1
  Constant_-1_e8c37/1 -> Product_08807/1
  Constant_x_qd_bdcc5/1 -> Subtract_9953e/1
  Constant_-1_5db2a/1 -> Product_e911c/1
  State_psi_q_SG_D_2_91656/1 -> Add_7b5f3/2
  Add_65cf9/1 -> Product_a83a1/2
  Product_7677e/1 -> Product_0e53f/1
  Product_08807/1 -> Add_bfdbe/1
  Constant_pi_184e6/1 -> Product_4e2f0/2
  Constant_f0_35b52/1 -> Product_0e53f/2
  Constant_x_qd_76623/1 -> Add_bfdbe/2
  State_psi_kq_SG_D_2_21fa1/1 -> Product_a70f7/1
  Subtract_9953e/1 -> Product_a70f7/2
  Product_e911c/1 -> Add_79dd5/1
  Input_v_q_SG_D_2_7d1d1/1 -> Product_f57b2/1
  Product_a83a1/1 -> Divide_28f81/1
  Product_0e53f/1 -> Divide_60bc7/2
  Add_bfdbe/1 -> Divide_28f81/2
  Product_a70f7/1 -> Divide_254b3/1
  Add_79dd5/1 -> Divide_254b3/2
  Divide_28f81/1 -> Subtract_651ed/1
  State_theta_SG_D_2_c47ee/1 -> MathFunc_cos_c1fb4/1
  Divide_254b3/1 -> Subtract_651ed/2
  Subtract_651ed/1 -> Add_7b5f3/1
  MathFunc_cos_c1fb4/1 -> Product_33a49/2
  Constant_R_a_e4cab/1 -> Product_4159f/1
  Add_7b5f3/1 -> Product_4159f/2
  State_theta_SG_D_2_7c757/1 -> MathFunc_sin_84ebb/1
  Product_4159f/1 -> Divide_7a6f1/1
  Product_4e2f0/1 -> Product_74126/1
  Product_f57b2/1 -> Subtract_e9756/2
  Constant_x_qdd_72180/1 -> Divide_7a6f1/2
  Input_v_d_SG_D_2_12f1d/1 -> Product_33a49/1
  Add_4d1a4/1 -> Product_2d533/2
  Divide_7a6f1/1 -> Subtract_52d26/1
  Product_33a49/1 -> Subtract_52d26/2
  MathFunc_sin_84ebb/1 -> Product_f57b2/2
  Product_2d533/1 -> Blockout_d_psi_q_SG_D_2_62d90/1
  State_psi_d_SG_D_2_b6b26/1 -> Product_2186e/1
  Constant_-2.0_8dfc0/1 -> Product_4e2f0/1
  Product_74126/1 -> Product_2d533/1
  Subtract_52d26/1 -> Subtract_e9756/1
  Product_2186e/1 -> Divide_60bc7/1
  Constant_f0_6845f/1 -> Product_74126/2
  Subtract_e9756/1 -> Add_4d1a4/1
  Divide_60bc7/1 -> Add_4d1a4/2

== system case7/SG_D_2/d_theta_SG_D_2_block ==
  note: d_theta_SG_D_2 in case7
      | $w_{\mathrm{SG},D,2}-2\,\pi \,f_{0}$
      | Automatically generated on 2025-10-31 19:24:46 .
  State_w_SG_D_2_14bd2 : Inport
  Add_e2fc1 : Sum
  Constant_-2.0_5e563 : Constant  Value=-2.0
  Constant_f0_f5ecd : Constant  Value=f0
  Constant_pi_bb70e : Constant  Value=pi
  Product_4db75 : Product
  Product_8ae60 : Product
  Blockout_d_theta_SG_D_2_87c37 : Outport
  wires:
  Constant_-2.0_5e563/1 -> Product_8ae60/1
  Constant_pi_bb70e/1 -> Product_8ae60/2
  Add_e2fc1/1 -> Blockout_d_theta_SG_D_2_87c37/1
  Product_8ae60/1 -> Product_4db75/1
  Constant_f0_f5ecd/1 -> Product_4db75/2
  Product_4db75/1 -> Add_e2fc1/1
  State_w_SG_D_2_14bd2/1 -> Add_e2fc1/2
